simulink model "Memdiode_1"  (R2019a)
settings: Solver=VariableStepAuto  StartTime=0.0  StopTime=200  MinStep=1e-30  RelTol=1e-2
model workspace (MAT data in the model file):
  I = Simulink.Signal
  I.DataType = 'auto'
  I.Dimensions = -1
  I.DimensionsMode = 'auto'
  I.Complexity = 'auto'
  I.SampleTime = -1
  I.SamplingMode = 'auto'
  I.InitialValue = '5.52082565263845e-06'
values from neighbouring files (symbols this model uses):
  amax = 1.7    [Simulink_memdiode.mat]
  amin = 1.5    [Simulink_memdiode.mat]
  etar = 60    [Simulink_memdiode.mat]
  etas = 100    [Simulink_memdiode.mat]
  Iomax = 0.0013    [Simulink_memdiode.mat]
  Iomin = 2.2e-05    [Simulink_memdiode.mat]
  Ri = 100    [Simulink_memdiode.mat]
  Rsmax = 117    [Simulink_memdiode.mat]
  Rsmin = 100    [Simulink_memdiode.mat]
  Vr = -1.5    [Simulink_memdiode.mat]
  Vs = 2.25    [Simulink_memdiode.mat]
libraries: simulink x1
settings Model: Creator=Barbats  LastModifiedBy=Barbats
settings SolverCC: ZeroCrossAlgorithm=Adaptive
settings OptimizationCC: BlockReduction=off  EfficientMapNaN2IntZero=off
settings HardwareCC: TargetBitPerPointer=64  TargetBitPerSizeT=64  TargetBitPerPtrDiffT=64  TargetLongLongMode=on  TargetIntDivRoundTo=Zero  TargetEndianess=LittleEndian  TargetWordSize=64  TargetHWDeviceType=MATLAB Host  ProdEqTarget=off
settings CodeAppCC: MaxIdLength=128
settings GRTTargetCC: TargetLangStandard=C89/C90 (ANSI)  GRTInterface=on

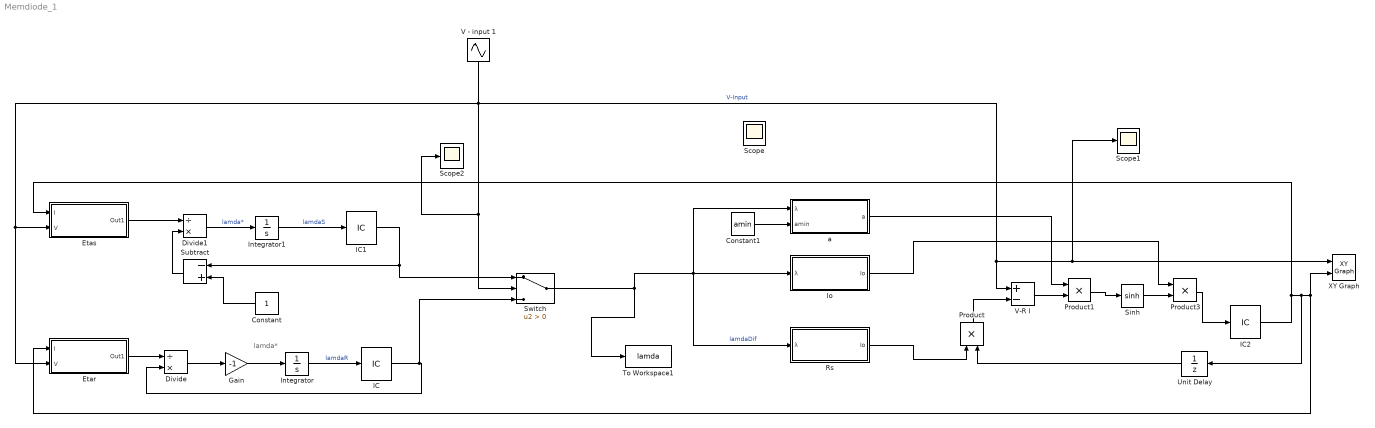
== system Memdiode_1 ==
  note: lamda*
  Constant : Constant
  Constant1 : Constant  Value=amin
  Divide : Product  Inputs=/*
  Divide1 : Product  Inputs=/*
  Etar : Subsystem
  Etas : Subsystem
  Gain : Gain  Gain=-1
  IC : InitialCondition
  IC1 : InitialCondition
  IC2 : InitialCondition  Value=1e-3
  Integrator : Integrator
  Integrator1 : Integrator
  Io : Subsystem
  Product : Product
  Product1 : Product
  Product3 : Product
  "Rs " : Subsystem
  Scope1 : Scope
  Scope2 : Scope
  Sinh : Trigonometry  Operator=sinh
  Subtract : Sum  Inputs=-+
  Switch : Switch  Criteria=u2 > Threshold
  To Workspace1 : ToWorkspace  VariableName=lamda  SampleTime=-1
  Unit Delay : UnitDelay  InitialCondition=5.52082565263845e-06  SampleTime=-1  HasFrameUpgradeWarning=on
  V - input 1 : Sin  Amplitude=2.5  Frequency=0.25  SampleTime=0
  V-R I : Sum  Inputs=+-
  XY Graph : simulink/Sinks/XY Graph  xmin=-3  xmax=3  ymin=-0.002  ymax=0.004  st=-1
  "a " : Subsystem
  Scope : Scope
  wires:
  V - input 1/1 -> Scope1/1, XY Graph/1, V-R I/1, Etas/2(V), Etar/2(V), Switch/2, Scope2/1  "V-Input"
  Product/1 -> V-R I/2
  Product1/1 -> Sinh/1
  Sinh/1 -> Product3/2
  V-R I/1 -> Product1/2
  "a "/1(a) -> Product1/1
  Io/1(Io) -> Product3/1
  "Rs "/1(Io) -> Product/1
  Integrator1/1 -> IC1/1  "lamdaS"
  Subtract/1 -> Divide1/2
  Divide1/1 -> Integrator1/1  "lamda*"
  Constant/1 -> Subtract/2
  Etas/1(Out1) -> Divide1/1
  IC1/1 -> Switch/1, Subtract/1
  Integrator/1 -> IC/1  "lamdaR"
  Etar/1(Out1) -> Divide/1
  Gain/1 -> Integrator/1
  Divide/1 -> Gain/1
  Switch/1 -> "Rs "/1(λ), Io/1(λ), "a "/1(λ), To Workspace1/1  "lamdaDif"
  Unit Delay/1 -> Product/2
  Product3/1 -> IC2/1
  IC/1 -> Switch/3, Divide/2
  Constant1/1 -> "a "/2(amin)
  IC2/1 -> Etas/1(I), XY Graph/2, Etar/1(I), Unit Delay/1

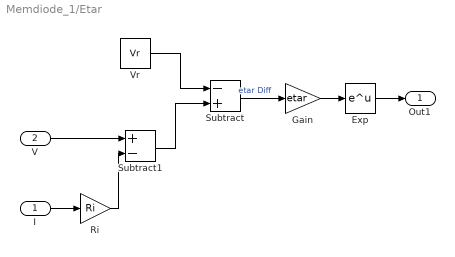
== system Memdiode_1/Etar ==
  I : Inport
  V : Inport  Port=2
  Exp : Math  SaturateOnIntegerOverflow=on
  Gain : Gain  Gain=etar
  "Ri " : Gain  Gain=Ri
  Subtract : Sum  Inputs=-+
  Subtract1 : Sum  Inputs=+-
  Vr : Constant  Value=Vr
  Out1 : Outport
  wires:
  Subtract1/1 -> Subtract/2
  Subtract/1 -> Gain/1  "etar Diff"
  Gain/1 -> Exp/1
  Exp/1 -> Out1/1
  I/1 -> "Ri "/1
  "Ri "/1 -> Subtract1/2
  Vr/1 -> Subtract/1
  V/1 -> Subtract1/1

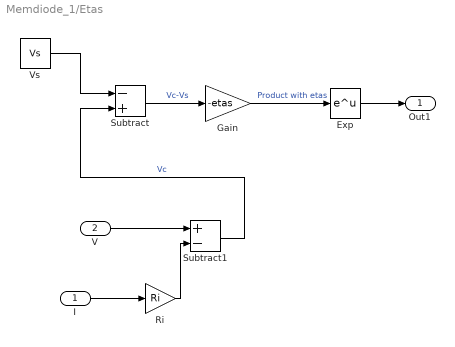
== system Memdiode_1/Etas ==
  I : Inport
  V : Inport  Port=2
  Exp : Math  SaturateOnIntegerOverflow=on
  Gain : Gain  Gain=-etas
  Ri : Gain  Gain=Ri
  Subtract : Sum  Inputs=-+
  Subtract1 : Sum  Inputs=+-
  Vs : Constant  Value=Vs
  Out1 : Outport
  wires:
  Vs/1 -> Subtract/1
  Subtract1/1 -> Subtract/2  "Vc"
  Gain/1 -> Exp/1  "Product with etas"
  Exp/1 -> Out1/1
  Ri/1 -> Subtract1/2
  I/1 -> Ri/1
  Subtract/1 -> Gain/1  "Vc-Vs"
  V/1 -> Subtract1/1

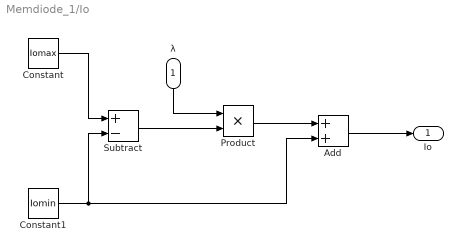
== system Memdiode_1/Io ==
  λ : Inport
  Add : Sum
  Constant : Constant  Value=Iomax
  Constant1 : Constant  Value=Iomin
  Product : Product
  Subtract : Sum  Inputs=+-
  Io : Outport
  wires:
  Constant/1 -> Subtract/1
  Constant1/1 -> Add/2, Subtract/2
  Subtract/1 -> Product/2
  λ/1 -> Product/1
  Product/1 -> Add/1
  Add/1 -> Io/1

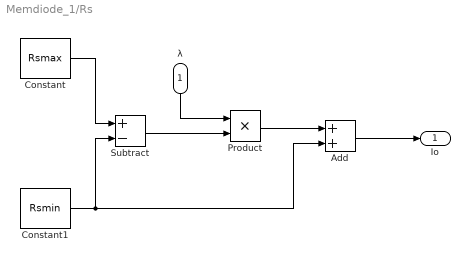
== system Memdiode_1/Rs  ==
  λ : Inport
  Add : Sum
  Constant : Constant  Value=Rsmax
  Constant1 : Constant  Value=Rsmin
  Product : Product
  Subtract : Sum  Inputs=+-
  Io : Outport
  wires:
  Constant/1 -> Subtract/1
  Constant1/1 -> Add/2, Subtract/2
  Subtract/1 -> Product/2
  λ/1 -> Product/1
  Product/1 -> Add/1
  Add/1 -> Io/1

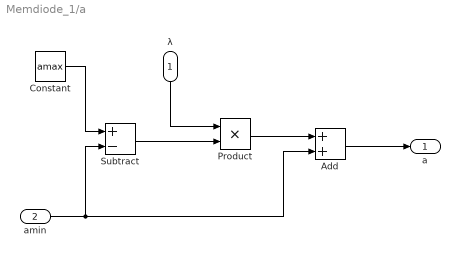
== system Memdiode_1/a  ==
  λ : Inport
  amin : Inport  Port=2
  Add : Sum
  Constant : Constant  Value=amax
  Product : Product
  Subtract : Sum  Inputs=+-
  a : Outport
  wires:
  Constant/1 -> Subtract/1
  amin/1 -> Add/2, Subtract/2
  Subtract/1 -> Product/2
  λ/1 -> Product/1
  Product/1 -> Add/1
  Add/1 -> a/1
